simulink model "hx_sim"  (R2017b)
settings: Solver=ode23tb  StartTime=0.0  StopTime=tEndSimul  MaxStep=0.1  RelTol=5e-6
values from neighbouring files (symbols this model uses):
  dnDt_in = mass_flow_converter(0.020, 'kg/min', 'mol/sec', 'Ammonia')    [hx.m]
  dnDt_out_liq = mass_flow_converter(0.020, 'kg/min', 'mol/sec', 'Ammonia')    [hx.m]
  dnDt_out_vap = mass_flow_converter(0, 'kg/h', 'mol/sec', 'Ammonia')    [hx.m]
  h_inner_liq = 1e2    (= 100)    [hx.m]
  h_inner_vap = 1e4    (= 10000)    [hx.m]
  h_outer = 200    [hx.m]
  L_min_water = 12.3    [hx.m]
  T_dnDt_in_C = 120    [hx.m]
  Tamb_C = 25    [hx.m]
  tEnd_dnDt_in = tStart_dnDt_in + 10 * c.min_to_sec    [hx.m]
  tEnd_dnDt_out_liq = tStart_dnDt_out_liq + 10 * c.min_to_sec    [hx.m]
  tEnd_dnDt_out_vap = tStart_dnDt_out_vap + 0 * c.min_to_sec    [hx.m]
  tStart_dnDt_in = 10 * c.min_to_sec    [hx.m]
  tStart_dnDt_out_liq = tEnd_dnDt_in + 5 * c.min_to_sec    [hx.m]
  tStart_dnDt_out_vap = 0    [hx.m]
  Twater_in_C = 20    [hx.m]
undefined symbols (not defined in the file or in its folder): h, P, T
libraries: thermochemical x11
settings Model: Creator=ferru  LastModifiedBy=fferrucc
settings SolverCC: AlgebraicLoopSolver=LineSearch

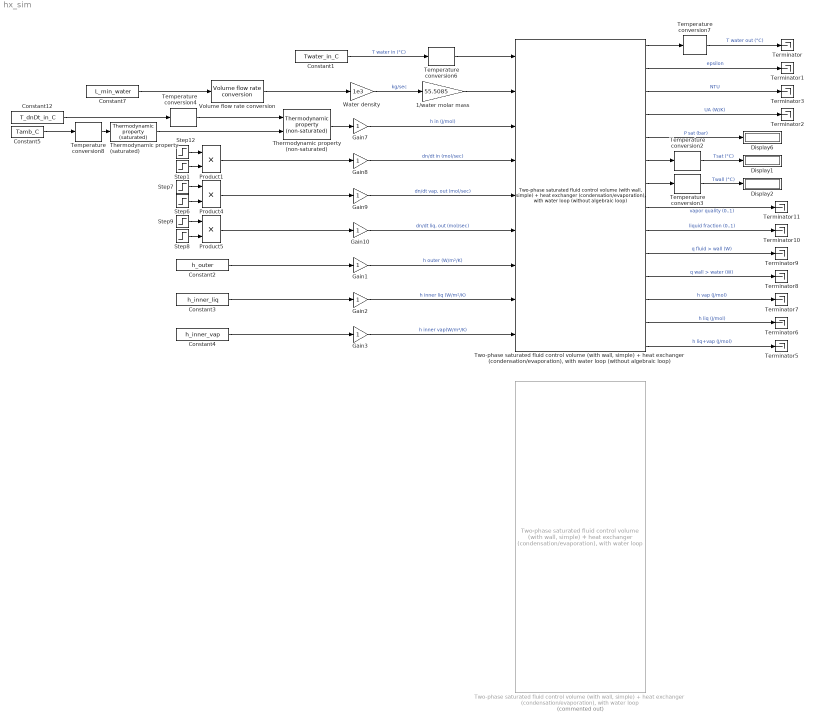
== system hx_sim ==
  1/water molar mass : Gain  Gain=55.5085
  Constant1 : Constant  Value=Twater_in_C
  Constant12 : Constant  Value=T_dnDt_in_C
  Constant2 : Constant  Value=h_outer
  Constant3 : Constant  Value=h_inner_liq
  Constant4 : Constant  Value=h_inner_vap
  Constant5 : Constant  Value=Tamb_C
  Constant7 : Constant  Value=L_min_water
  Display1 : Display
  Display2 : Display
  Display6 : Display
  Gain{1..3,7..10} (7 alike) : Gain
  Product1 : Product
  Product4 : Product
  Product5 : Product
  Step1 : Step  Time=tEnd_dnDt_in  Before=1  After=0  SampleTime=0
  Step12 : Step  Time=tStart_dnDt_in  After=dnDt_in  SampleTime=0
  Step6 : Step  Time=tEnd_dnDt_out_vap  Before=1  After=0  SampleTime=0
  Step7 : Step  Time=tStart_dnDt_out_vap  After=dnDt_out_vap  SampleTime=0
  Step8 : Step  Time=tEnd_dnDt_out_liq  Before=1  After=0  SampleTime=0
  Step9 : Step  Time=tStart_dnDt_out_liq  After=dnDt_out_liq  SampleTime=0
  Temperature conversion2 : thermochemical/Conversions/Temperature conversion  sel=K --> °C
      settings: SourceProductName=@ Thermochemical
  Temperature conversion3 : thermochemical/Conversions/Temperature conversion  sel=K --> °C
      settings: SourceProductName=@ Thermochemical
  Temperature conversion4 : thermochemical/Conversions/Temperature conversion  sel=°C --> K
      settings: SourceProductName=@ Thermochemical
  Temperature conversion6 : thermochemical/Conversions/Temperature conversion  sel=°C --> K
      settings: SourceProductName=@ Thermochemical
  Temperature conversion7 : thermochemical/Conversions/Temperature conversion  sel=K --> °C
      settings: SourceProductName=@ Thermochemical
  Temperature conversion8 : thermochemical/Conversions/Temperature conversion  sel=°C --> K
      settings: SourceProductName=@ Thermochemical
  Terminator{,1..3,5..11} (11 alike) : Terminator
  Thermodynamic property (non-saturated) : thermochemical/Thermodynamic fluid properties/Thermodynamic  property (non-saturated)  sel=h(T,P)  fluid=fluid  reciprocVar=-1  lookup2D_BreakPoint1=fluid.no_sat.T_P_indep.var_indep.T  lookup2D_BreakPoint2=fluid.no_sat.T_P_indep.var_indep.P  lookup2D_Data=fluid.no_sat.T_P_indep.var_dep.h_molar
      settings: SourceProductName=@ Thermochemical
  Thermodynamic property (saturated) : thermochemical/Thermodynamic fluid properties/Thermodynamic  property (saturated)  sel=P(T) (bar)  fluid=fluid  lookup1D_BreakPoint1=fluid.sat.T  lookup1D_Data=fluid.sat.Psat
      settings: SourceProductName=@ Thermochemical
  "Two-phase saturated fluid control volume (with wall, simple) + heat exchanger (condensation/evaporation), with water loop" : thermochemical/Control volumes/Two-phase saturated fluid control volume (with wall, simple) + heat exchanger (condensation//evaporation), with water loop  Commented=on
      link override "Two-phase saturated fluid control volume (with wall, simple)/Two-phase saturated fluid control volume (without walls)": N_init=Nhx_init  T_init=Thx_init  V=Vhx
      link override "Two-phase saturated fluid control volume (with wall, simple)/Wall, simple, h as inputs": material=Stainless steel AISI316  cp=490.8  rho=8023  s=Shx_m2  e_mm=thickness_hx_mm  mass=2.2529
      settings: SourceProductName=@ Thermochemical
  "Two-phase saturated fluid control volume (with wall, simple) + heat exchanger (condensation/evaporation), with water loop (without algebraic loop)" : thermochemical/Control volumes/Two-phase saturated fluid control volume (with wall, simple) + heat exchanger (condensation//evaporation), with water loop (without algebraic loop)
      link override "Two-phase saturated fluid control volume (with wall, simple) (without algebraic loop)/Two-phase saturated fluid control volume (without walls) (without algebraic loop)": N_init=Nhx_init  T_init=Thx_init  V=Vhx
      link override "Two-phase saturated fluid control volume (with wall, simple) (without algebraic loop)/Wall, simple, h as inputs": material=Stainless steel AISI316  cp=490.8  rho=8023  s=Shx_m2  e_mm=thickness_hx_mm  mass=2.2529  Twall_init=Thx_init
      settings: SourceProductName=@ Thermochemical
  Volume flow rate conversion : thermochemical/Conversions/Volume flow rate conversion  sel=L/min --> m3/sec
      settings: SourceProductName=@ Thermochemical
  Water density : Gain  Gain=1e3
  wires:
  Step12/1 -> Product1/1
  Step1/1 -> Product1/2
  Constant12/1 -> Temperature conversion4/1
  Temperature conversion4/1 -> Thermodynamic property (non-saturated)/1
  Temperature conversion2/1 -> Display1/1  "Tsat (°C)"
  "Two-phase saturated fluid control volume (with wall, simple) + heat exchanger (condensation/evaporation), with water loop (without algebraic loop)"/6 -> Temperature conversion2/1
  Gain7/1 -> "Two-phase saturated fluid control volume (with wall, simple) + heat exchanger (condensation/evaporation), with water loop (without algebraic loop)"/3  "h in (J/mol)"
  Gain8/1 -> "Two-phase saturated fluid control volume (with wall, simple) + heat exchanger (condensation/evaporation), with water loop (without algebraic loop)"/4  "dn/dt in (mol/sec)"
  Gain9/1 -> "Two-phase saturated fluid control volume (with wall, simple) + heat exchanger (condensation/evaporation), with water loop (without algebraic loop)"/5  "dn/dt vap, out (mol/sec)"
  Gain10/1 -> "Two-phase saturated fluid control volume (with wall, simple) + heat exchanger (condensation/evaporation), with water loop (without algebraic loop)"/6  "dn/dt liq, out (mol/sec)"
  "Two-phase saturated fluid control volume (with wall, simple) + heat exchanger (condensation/evaporation), with water loop (without algebraic loop)"/5 -> Display6/1  "P sat (bar)"
  "Two-phase saturated fluid control volume (with wall, simple) + heat exchanger (condensation/evaporation), with water loop (without algebraic loop)"/9 -> Terminator10/1  "liquid fraction (0..1)"
  "Two-phase saturated fluid control volume (with wall, simple) + heat exchanger (condensation/evaporation), with water loop (without algebraic loop)"/8 -> Terminator11/1  "vapor quality (0..1)"
  "Two-phase saturated fluid control volume (with wall, simple) + heat exchanger (condensation/evaporation), with water loop (without algebraic loop)"/12 -> Terminator7/1  "h vap (J/mol)"
  "Two-phase saturated fluid control volume (with wall, simple) + heat exchanger (condensation/evaporation), with water loop (without algebraic loop)"/14 -> Terminator5/1  "h liq+vap (J/mol)"
  "Two-phase saturated fluid control volume (with wall, simple) + heat exchanger (condensation/evaporation), with water loop (without algebraic loop)"/13 -> Terminator6/1  "h liq (J/mol)"
  Constant1/1 -> Temperature conversion6/1  "T water in (°C)"
  Thermodynamic property (non-saturated)/1 -> Gain7/1
  Product1/1 -> Gain8/1
  Product4/1 -> Gain9/1
  Step6/1 -> Product4/2
  Step7/1 -> Product4/1
  Step9/1 -> Product5/1
  Step8/1 -> Product5/2
  Product5/1 -> Gain10/1
  "Two-phase saturated fluid control volume (with wall, simple) + heat exchanger (condensation/evaporation), with water loop (without algebraic loop)"/7 -> Temperature conversion3/1
  Temperature conversion3/1 -> Display2/1  "Twall (°C)"
  "Two-phase saturated fluid control volume (with wall, simple) + heat exchanger (condensation/evaporation), with water loop (without algebraic loop)"/11 -> Terminator8/1  "q wall > water (W)"
  "Two-phase saturated fluid control volume (with wall, simple) + heat exchanger (condensation/evaporation), with water loop (without algebraic loop)"/10 -> Terminator9/1  "q fluid > wall (W)"
  Temperature conversion7/1 -> Terminator/1  "T water out (°C)"
  Gain3/1 -> "Two-phase saturated fluid control volume (with wall, simple) + heat exchanger (condensation/evaporation), with water loop (without algebraic loop)"/9  "h inner vap(W/m²/K)"
  Gain1/1 -> "Two-phase saturated fluid control volume (with wall, simple) + heat exchanger (condensation/evaporation), with water loop (without algebraic loop)"/7  "h outer (W/m²/K)"
  Gain2/1 -> "Two-phase saturated fluid control volume (with wall, simple) + heat exchanger (condensation/evaporation), with water loop (without algebraic loop)"/8  "h inner liq (W/m²/K)"
  Constant2/1 -> Gain1/1
  Constant3/1 -> Gain2/1
  Constant4/1 -> Gain3/1
  Constant5/1 -> Temperature conversion8/1
  Temperature conversion8/1 -> Thermodynamic property (saturated)/1
  Thermodynamic property (saturated)/1 -> Thermodynamic property (non-saturated)/2
  Temperature conversion6/1 -> "Two-phase saturated fluid control volume (with wall, simple) + heat exchanger (condensation/evaporation), with water loop (without algebraic loop)"/1
  Volume flow rate conversion/1 -> Water density/1
  1/water molar mass/1 -> "Two-phase saturated fluid control volume (with wall, simple) + heat exchanger (condensation/evaporation), with water loop (without algebraic loop)"/2
  Water density/1 -> 1/water molar mass/1  "kg/sec"
  Constant7/1 -> Volume flow rate conversion/1
  "Two-phase saturated fluid control volume (with wall, simple) + heat exchanger (condensation/evaporation), with water loop (without algebraic loop)"/4 -> Terminator2/1  "UA (W/K)"
  "Two-phase saturated fluid control volume (with wall, simple) + heat exchanger (condensation/evaporation), with water loop (without algebraic loop)"/3 -> Terminator3/1  "NTU"
  "Two-phase saturated fluid control volume (with wall, simple) + heat exchanger (condensation/evaporation), with water loop (without algebraic loop)"/1 -> Temperature conversion7/1
  "Two-phase saturated fluid control volume (with wall, simple) + heat exchanger (condensation/evaporation), with water loop (without algebraic loop)"/2 -> Terminator1/1  "epsilon"
